simulink model "quadrotor"  (R2022b)
settings: Solver=ode4  StartTime=0.0  StopTime=120  FixedStep=0.01  RelTol=1e-3
InitFcn:
  | initial_conditions_and_parameters;
values from neighbouring files (symbols this model uses):
  ang_max = 6*pi/180    (= 0.10471975512)    [initial_conditions_and_parameters.m]
  CD = [0.018944 0.018944 0.018944]    [initial_conditions_and_parameters.m]
  data = zeros(data_len,1)    [initial_conditions_and_parameters.m]
  delay_a = 0    [initial_conditions_and_parameters.m]
  delay_sample = 0.1    [initial_conditions_and_parameters.m]
  delay_v = 0.1    [initial_conditions_and_parameters.m]
  ESC_k = 718.078    [initial_conditions_and_parameters.m]
  ESC_p = 88.448    [initial_conditions_and_parameters.m]
  f_g = [0 0 0]    [initial_conditions_and_parameters.m]
  ftau_b = [0 0 0]    [initial_conditions_and_parameters.m]
  g = 9.8    [initial_conditions_and_parameters.m]
  hM = 1.982e-7    (= 1.982e-07)    [initial_conditions_and_parameters.m]
  hT = 1.239e-5    (= 1.239e-05)    [initial_conditions_and_parameters.m]
  Ir = 3.789e-6    (= 3.789e-06)    [initial_conditions_and_parameters.m]
  Ix = 0.01    [initial_conditions_and_parameters.m]
  Iy = 0.01    [initial_conditions_and_parameters.m]
  Iz = 0.02    [initial_conditions_and_parameters.m]
  kd_phi = 70    [initial_conditions_and_parameters.m]
  kd_psi = 70    [initial_conditions_and_parameters.m]
  kd_theta = 70    [initial_conditions_and_parameters.m]
  kd_x = 1    [initial_conditions_and_parameters.m]
  kd_y = 1    [initial_conditions_and_parameters.m]
  kd_z = 1    [initial_conditions_and_parameters.m]
  Kdphi_D = 0.03    [initial_conditions_and_parameters.m]
  Kdphi_I = 0.68    [initial_conditions_and_parameters.m]
  Kdphi_P = 1    [initial_conditions_and_parameters.m]
  Kdpsi_D = 0.03    [initial_conditions_and_parameters.m]
  Kdpsi_I = 0.68    [initial_conditions_and_parameters.m]
  Kdpsi_P = 1    [initial_conditions_and_parameters.m]
  Kdtheta_D = 0.03    [initial_conditions_and_parameters.m]
  Kdtheta_I = 0.68    [initial_conditions_and_parameters.m]
  Kdtheta_P = 1    [initial_conditions_and_parameters.m]
  kp_phi = 250    [initial_conditions_and_parameters.m]
  kp_psi = 250    [initial_conditions_and_parameters.m]
  kp_theta = 250    [initial_conditions_and_parameters.m]
  kp_x = 0    [initial_conditions_and_parameters.m]
  kp_y = 0    [initial_conditions_and_parameters.m]
  kp_z = 20    [initial_conditions_and_parameters.m]
  Kvx_D = 0.15    [initial_conditions_and_parameters.m]
  Kvx_I = 0.1    [initial_conditions_and_parameters.m]
  Kvx_P = 0.3    [initial_conditions_and_parameters.m]
  Kvy_D = 0.15    [initial_conditions_and_parameters.m]
  Kvy_I = 0.1    [initial_conditions_and_parameters.m]
  Kvy_P = 0.3    [initial_conditions_and_parameters.m]
  Kvz_D = 0    [initial_conditions_and_parameters.m]
  Kvz_I = 0.1    [initial_conditions_and_parameters.m]
  Kvz_P = 1    [initial_conditions_and_parameters.m]
  LT = 0.1*sqrt(2)    [initial_conditions_and_parameters.m]
  m = 0.5    [initial_conditions_and_parameters.m]
  noise_a = 0.0005    [initial_conditions_and_parameters.m]
  noise_v = 0.0015    [initial_conditions_and_parameters.m]
  p_initial = 0    [initial_conditions_and_parameters.m]
  phi_initial = 0    [initial_conditions_and_parameters.m]
  psi_initial = 0    [initial_conditions_and_parameters.m]
  q_initial = 0    [initial_conditions_and_parameters.m]
  r_initial = 0    [initial_conditions_and_parameters.m]
  sample_a = 0.01    [initial_conditions_and_parameters.m]
  sample_v = 0.04    [initial_conditions_and_parameters.m]
  seed_delay_phi = floor(rand()*10000000)    [initial_conditions_and_parameters.m]
  seed_delay_psi = floor(rand()*10000000)    [initial_conditions_and_parameters.m]
  seed_delay_theta = floor(rand()*10000000)    [initial_conditions_and_parameters.m]
  seed_delay_vx = floor(rand()*10000000)    [initial_conditions_and_parameters.m]
  seed_delay_vy = floor(rand()*10000000)    [initial_conditions_and_parameters.m]
  seed_delay_vz = floor(rand()*10000000)    [initial_conditions_and_parameters.m]
  seed_phi = floor(rand()*10000000)    [initial_conditions_and_parameters.m]
  seed_psi = floor(rand()*10000000)    [initial_conditions_and_parameters.m]
  seed_theta = floor(rand()*10000000)    [initial_conditions_and_parameters.m]
  seed_vx = floor(rand()*10000000)    [initial_conditions_and_parameters.m]
  seed_vy = floor(rand()*10000000)    [initial_conditions_and_parameters.m]
  seed_vz = floor(rand()*10000000)    [initial_conditions_and_parameters.m]
  sweep_amp = 1    [main.m]
  T_max = 30    [initial_conditions_and_parameters.m]
  tau_x_max = 1    [initial_conditions_and_parameters.m]
  tau_y_max = 1    [initial_conditions_and_parameters.m]
  tau_z_max = 1    [initial_conditions_and_parameters.m]
  theta_initial = 0    [initial_conditions_and_parameters.m]
  u_initial = 0    [initial_conditions_and_parameters.m]
  v_initial = 0    [initial_conditions_and_parameters.m]
  w_initial = 0    [initial_conditions_and_parameters.m]
  x_g_initial = 0    [initial_conditions_and_parameters.m]
  y_g_initial = 0    [initial_conditions_and_parameters.m]
  z_g_initial = 0    [initial_conditions_and_parameters.m]
libraries: simulink x12
settings Model: Creator=Sky  LastModifiedBy=xpp
settings SolverCC: AlgebraicLoopSolver=LineSearch
settings DataIOCC: SignalLogging=off
settings DebuggingCC: InheritedTsInSrcMsg=none  TasksWithSamePriorityMsg=none  SigSpecEnsureSampleTimeMsg=none  UnconnectedInputMsg=warning  UnconnectedOutputMsg=warning  UnconnectedLineMsg=warning  UnknownTsInhSupMsg=none  SFMachineParentedDataDiag=warning  ArithmeticOperatorsInVariantConditions=warning
settings ModelReferenceCC: EnableRefExpFcnMdlSchedulingChecks=on
settings SFSimCC: SimUseLocalCustomCode=off  CustomCodeUndefinedFunction=UseInterfaceOnly
settings RTWCC: RTWUseLocalCustomCode=off  DLArmComputeVersion=19.05

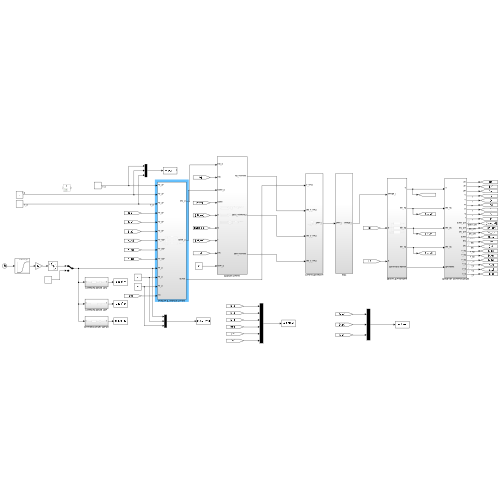
[thumbnail: Simulink's stored preview of the top-level diagram]
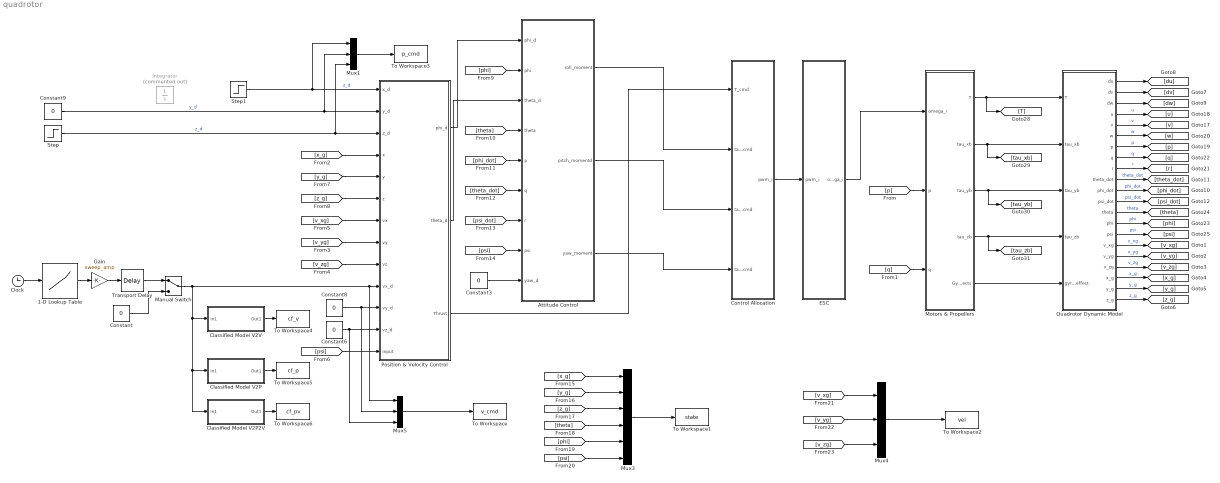
== system quadrotor ==
  1-D Lookup Table : Lookup_n-D  NumberOfTableDimensions=1  BreakpointsForDimension1=t  Table=data  InternalRulePriority=Speed  RndMeth=Simplest
  Attitude Control : Subsystem
  Classified Model V2P : Subsystem
  Classified Model V2P2V : Subsystem
  Classified Model V2V : Subsystem
  Clock : Clock
  Constant : Constant  Value=0
  Constant3 : Constant  Value=0
  Constant6 : Constant  Value=0  SampleTime=-1
  Constant8 : Constant  Value=0  SampleTime=-1
  Constant9 : Constant  Value=0  SampleTime=-1
  Control Allocation : Subsystem
  ESC : Subsystem
  Gain : Gain  Gain=sweep_amp
  Integrator : Integrator  Commented=on
  Manual Switch : ManualSwitch
  Motors & Propellers : Subsystem
  Mux1 : Mux  Inputs=3
  Mux3 : Mux  Inputs=6
  Mux4 : Mux  Inputs=3
  Mux5 : Mux  Inputs=3
  Position & Velocity Control : Subsystem
  Quadrotor Dynamic Model : Subsystem
  Step : Step  SampleTime=0
  Step1 : Step  Time=20  SampleTime=0
  To Workspace : ToWorkspace  VariableName=v_cmd  SampleTime=-1
      settings: Save2DSignal=2-D array (concatenate along first dimension)
  To Workspace1 : ToWorkspace  VariableName=state  SampleTime=-1
      settings: Save2DSignal=2-D array (concatenate along first dimension)
  To Workspace2 : ToWorkspace  VariableName=vel  SampleTime=-1
      settings: Save2DSignal=2-D array (concatenate along first dimension)
  To Workspace3 : ToWorkspace  VariableName=p_cmd  SampleTime=-1
      settings: Save2DSignal=2-D array (concatenate along first dimension)
  To Workspace4 : ToWorkspace  VariableName=cf_v  SampleTime=-1
      settings: Save2DSignal=2-D array (concatenate along first dimension)
  To Workspace5 : ToWorkspace  VariableName=cf_p  SampleTime=-1
      settings: Save2DSignal=2-D array (concatenate along first dimension)
  To Workspace6 : ToWorkspace  VariableName=cf_pv  SampleTime=-1
      settings: Save2DSignal=2-D array (concatenate along first dimension)
  Transport Delay : TransportDelay  DelayTime=20  BufferSize=4096
  wires:
  [q] -> Motors & Propellers/3(q)
  [p] -> Motors & Propellers/2(p)
  Motors & Propellers/1(T) -> Quadrotor Dynamic Model/1(T), [T]
  Motors & Propellers/2(tau_xb) -> Quadrotor Dynamic Model/2(tau_xb), [tau_xb]
  Motors & Propellers/3(tau_yb) -> Quadrotor Dynamic Model/3(tau_yb), [tau_yb]
  Motors & Propellers/4(tau_zb) -> Quadrotor Dynamic Model/4(tau_zb), [tau_zb]
  Quadrotor Dynamic Model/3(dw) -> [dw]
  Quadrotor Dynamic Model/8(q) -> [q]  "q"
  Quadrotor Dynamic Model/12(psi_dot) -> [psi_dot]  "psi_dot"
  Quadrotor Dynamic Model/18(v_zg) -> [v_zg]  "v_zg"
  Quadrotor Dynamic Model/5(v) -> [v]  "v"
  Quadrotor Dynamic Model/9(r) -> [r]  "r"
  Quadrotor Dynamic Model/11(phi_dot) -> [phi_dot]  "phi_dot"
  Quadrotor Dynamic Model/1(du) -> [du]
  Quadrotor Dynamic Model/19(x_g) -> [x_g]  "x_g"
  Quadrotor Dynamic Model/20(y_g) -> [y_g]  "y_g"
  Quadrotor Dynamic Model/16(v_xg) -> [v_xg]  "v_xg"
  Quadrotor Dynamic Model/15(psi) -> [psi]  "psi"
  Quadrotor Dynamic Model/4(u) -> [u]  "u"
  Quadrotor Dynamic Model/13(theta) -> [theta]  "theta"
  Quadrotor Dynamic Model/17(v_yg) -> [v_yg]  "v_yg"
  Quadrotor Dynamic Model/14(phi) -> [phi]  "phi"
  Quadrotor Dynamic Model/21(z_g) -> [z_g]  "z_g"
  Quadrotor Dynamic Model/6(w) -> [w]  "w"
  Quadrotor Dynamic Model/7(p) -> [p]  "p"
  Quadrotor Dynamic Model/2(dv) -> [dv]
  Quadrotor Dynamic Model/10(theta_dot) -> [theta_dot]  "theta_dot"
  [x_g] -> Position & Velocity Control/4(x)
  [v_yg] -> Position & Velocity Control/8(vy)
  [v_zg] -> Position & Velocity Control/9(vz)
  [v_xg] -> Position & Velocity Control/7(vx)
  [y_g] -> Position & Velocity Control/5(y)
  [z_g] -> Position & Velocity Control/6(z)
  Position & Velocity Control/1(phi_d) -> Attitude Control/1(phi_d)
  Position & Velocity Control/2(theta_d) -> Attitude Control/3(theta_d)
  [phi] -> Attitude Control/2(phi)
  [theta] -> Attitude Control/4(theta)
  [phi_dot] -> Attitude Control/5(p)
  [theta_dot] -> Attitude Control/6(q)
  [psi_dot] -> Attitude Control/7(r)
  [psi] -> Attitude Control/8(psi)
  Constant9/1 -> Mux1/2, Position & Velocity Control/2(y_d)  "y_d"
  Step/1 -> Mux1/3, Position & Velocity Control/3(z_d)  "z_d"
  Constant3/1 -> Attitude Control/9(yaw_d)
  Control Allocation/1(pwm_i) -> ESC/1(pwm_i)
  ESC/1(omega_i) -> Motors & Propellers/1(omega_i)
  Attitude Control/3(yaw_moment) -> Control Allocation/4(tau_z_cmd)
  Attitude Control/1(roll_moment) -> Control Allocation/2(tau_x_cmd)
  Attitude Control/2(pitch_momentd) -> Control Allocation/3(tau_y_cmd)
  Position & Velocity Control/3(Thrust) -> Control Allocation/1(T_cmd)
  Motors & Propellers/5(Gyroscopic effects) -> Quadrotor Dynamic Model/5(gyroeffect)
  Mux3/1 -> To Workspace1/1
  [x_g] -> Mux3/1
  [y_g] -> Mux3/2
  [z_g] -> Mux3/3
  [theta] -> Mux3/4
  [phi] -> Mux3/5
  [psi] -> Mux3/6
  Mux5/1 -> To Workspace/1
  Constant6/1 -> Mux5/3, Position & Velocity Control/12(vz_d)
  Constant8/1 -> Mux5/2, Position & Velocity Control/11(vy_d)
  Clock/1 -> 1-D Lookup Table/1
  Mux4/1 -> To Workspace2/1
  [v_zg] -> Mux4/3
  [v_yg] -> Mux4/2
  [v_xg] -> Mux4/1
  Step1/1 -> Mux1/1, Position & Velocity Control/1(x_d)  "z_d"
  Mux1/1 -> To Workspace3/1
  [psi] -> Position & Velocity Control/13(Input)
  Manual Switch/1 -> Classified Model V2P2V/1(In1), Classified Model V2P/1(In1), Classified Model V2V/1(In1), Mux5/1, Position & Velocity Control/10(vx_d)
  Transport Delay/1 -> Manual Switch/1
  Constant/1 -> Manual Switch/2
  Classified Model V2V/1(Out1) -> To Workspace4/1
  Classified Model V2P/1(Out1) -> To Workspace5/1
  Classified Model V2P2V/1(Out1) -> To Workspace6/1
  Gain/1 -> Transport Delay/1
  1-D Lookup Table/1 -> Gain/1

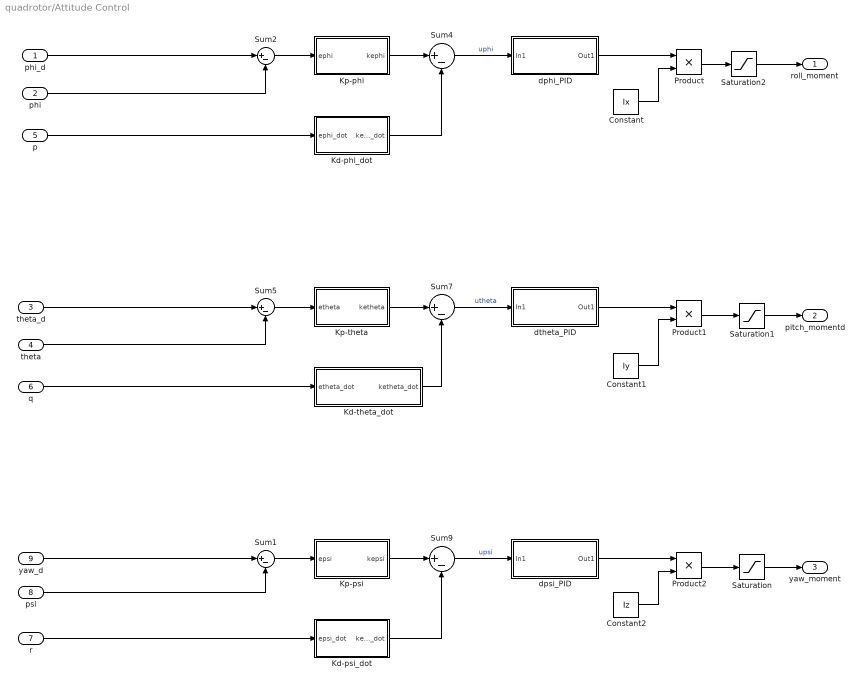
== system quadrotor/Attitude Control ==
  phi_d : Inport
  phi : Inport  Port=2
  theta_d : Inport  Port=3
  theta : Inport  Port=4
  p : Inport  Port=5
  q : Inport  Port=6
  r : Inport  Port=7
  psi : Inport  Port=8
  yaw_d : Inport  Port=9
  Constant : Constant  Value=Ix
  Constant1 : Constant  Value=Iy
  Constant2 : Constant  Value=Iz
  Kd-phi_dot : Subsystem
  Kd-psi_dot : Subsystem
  Kd-theta_dot : Subsystem
  Kp-phi : Subsystem
  Kp-psi : Subsystem
  Kp-theta : Subsystem
  Product : Product  OutMin=[-1]  OutMax=[1]
  Product1 : Product  OutMin=[-1]  OutMax=[1]
  Product2 : Product  OutMin=[-1]  OutMax=[1]
  Saturation : Saturate  UpperLimit=tau_z_max  LowerLimit=-tau_z_max
  Saturation1 : Saturate  UpperLimit=tau_y_max  LowerLimit=-tau_y_max
  Saturation2 : Saturate  UpperLimit=tau_x_max  LowerLimit=-tau_x_max
  Sum{1..2,4..5,7,9} (6 alike) : Sum  Inputs=|+-
  dphi_PID : Subsystem
  dpsi_PID : Subsystem
  dtheta_PID : Subsystem
  roll_moment : Outport
  pitch_momentd : Outport  Port=2
  yaw_moment : Outport  Port=3
  wires:
  r/1 -> Kd-psi_dot/1(epsi_dot)
  Sum1/1 -> Kp-psi/1(epsi)
  p/1 -> Kd-phi_dot/1(ephi_dot)
  Sum2/1 -> Kp-phi/1(ephi)
  phi_d/1 -> Sum2/1
  Kd-phi_dot/1(kephi_dot) -> Sum4/2
  q/1 -> Kd-theta_dot/1(etheta_dot)
  Sum5/1 -> Kp-theta/1(etheta)
  theta_d/1 -> Sum5/1
  Kd-theta_dot/1(ketheta_dot) -> Sum7/2
  yaw_d/1 -> Sum1/1
  Constant/1 -> Product/2
  Product/1 -> Saturation2/1
  Product1/1 -> Saturation1/1
  Constant1/1 -> Product1/2
  Product2/1 -> Saturation/1
  Constant2/1 -> Product2/2
  Saturation/1 -> yaw_moment/1
  Saturation1/1 -> pitch_momentd/1
  Saturation2/1 -> roll_moment/1
  Kp-phi/1(kephi) -> Sum4/1
  Kp-theta/1(ketheta) -> Sum7/1
  Kp-psi/1(kepsi) -> Sum9/1
  Kd-psi_dot/1(kepsi_dot) -> Sum9/2
  dphi_PID/1(Out1) -> Product/1
  Sum4/1 -> dphi_PID/1(In1)  "uphi"
  Sum7/1 -> dtheta_PID/1(In1)  "utheta"
  dtheta_PID/1(Out1) -> Product1/1
  Sum9/1 -> dpsi_PID/1(In1)  "upsi"
  dpsi_PID/1(Out1) -> Product2/1
  phi/1 -> Sum2/2
  theta/1 -> Sum5/2
  psi/1 -> Sum1/2

== system quadrotor/Classified Model V2P ==
  In1 : Inport
  Transfer Fcn : TransferFcn  Numerator=[2.218]  Denominator=[1 2.1565 0.0006694]
  Transport Delay : TransportDelay  DelayTime=0.06
  Out1 : Outport
  wires:
  Transfer Fcn/1 -> Transport Delay/1
  In1/1 -> Transfer Fcn/1
  Transport Delay/1 -> Out1/1

== system quadrotor/Classified Model V2P2V ==
  In1 : Inport
  Transfer Fcn : TransferFcn  Numerator=[2.218]  Denominator=[1 2.16]
  Transport Delay : TransportDelay  DelayTime=0.06
  Out1 : Outport
  wires:
  Transfer Fcn/1 -> Transport Delay/1
  In1/1 -> Transfer Fcn/1
  Transport Delay/1 -> Out1/1

== system quadrotor/Classified Model V2V ==
  In1 : Inport
  Transfer Fcn : TransferFcn  Numerator=[2.135]  Denominator=[1 2.016]
  Transport Delay : TransportDelay  DelayTime=0.06
  Out1 : Outport
  wires:
  In1/1 -> Transfer Fcn/1
  Transfer Fcn/1 -> Transport Delay/1
  Transport Delay/1 -> Out1/1

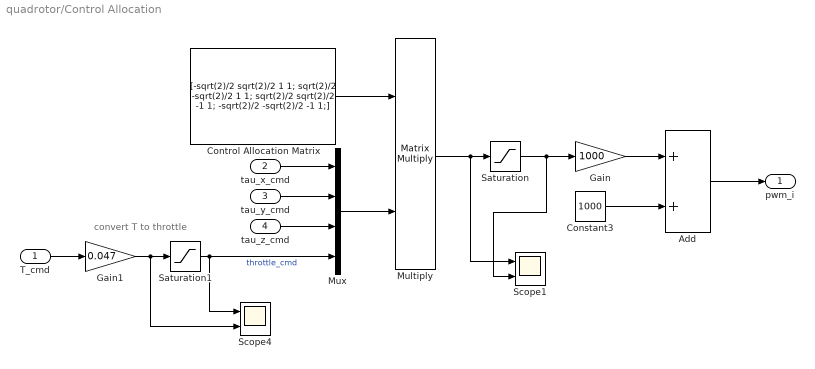
== system quadrotor/Control Allocation ==
  note: convert T to throttle
  T_cmd : Inport
  tau_x_cmd : Inport  Port=2
  tau_y_cmd : Inport  Port=3
  tau_z_cmd : Inport  Port=4
  Add : Sum
  Constant3 : Constant  Value=1000
  Control Allocation Matrix : Constant  Value="[-sqrt(2)/2  sqrt(2)/2  1 1; sqrt(2)/2 -sqrt(2)/2  1 1; sqrt(2)/2  sqrt(2)/2 -1 1; -sqrt(2)/2 -sqrt(2)/2 -1 1;]"
  Gain : Gain  Gain=1000  OutDataTypeStr=Inherit: Same as input
  Gain1 : Gain  Gain=0.047
  Multiply : Product  Multiplication=Matrix(*)  OutDataTypeStr=Inherit: Same as first input
  Mux : Mux
  Saturation : Saturate  UpperLimit=1  LowerLimit=0
  Saturation1 : Saturate  UpperLimit=1  LowerLimit=0
  Scope1 : Scope  NumInputPorts=2
  Scope4 : Scope  NumInputPorts=2
  pwm_i : Outport  VectorParamsAs1DForOutWhenUnconnected=off
  wires:
  Constant3/1 -> Add/2
  Saturation/1 -> Scope1/2, Gain/1
  Saturation1/1 -> Scope4/1, Mux/4  "throttle_cmd"
  tau_y_cmd/1 -> Mux/2
  Add/1 -> pwm_i/1
  Multiply/1 -> Scope1/1, Saturation/1
  Gain/1 -> Add/1
  tau_x_cmd/1 -> Mux/1
  tau_z_cmd/1 -> Mux/3
  Mux/1 -> Multiply/2
  Control Allocation Matrix/1 -> Multiply/1
  Gain1/1 -> Scope4/2, Saturation1/1
  T_cmd/1 -> Gain1/1

== system quadrotor/ESC ==
  pwm_i : Inport
  Add : Sum  AccumDataTypeStr=double
  Constant : Constant  Value=ESC_p
  Constant3 : Constant  Value=1000  OutDataTypeStr=double
  Gain : Gain  Gain=0.001  OutDataTypeStr=Inherit: Same as input
  Gain1 : Gain  Gain=ESC_k  OutDataTypeStr=Inherit: Same as input
  Saturation : Saturate  UpperLimit=2000  LowerLimit=1000
  Sum : Sum  Inputs=|+-
  omega_i : Outport  VectorParamsAs1DForOutWhenUnconnected=off
  wires:
  Constant3/1 -> Sum/2
  pwm_i/1 -> Saturation/1
  Saturation/1 -> Sum/1
  Sum/1 -> Gain/1
  Constant/1 -> Add/2
  Gain/1 -> Gain1/1
  Gain1/1 -> Add/1
  Add/1 -> omega_i/1

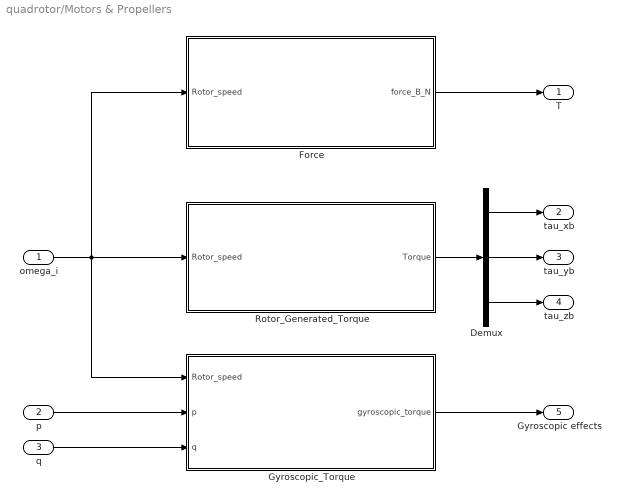
== system quadrotor/Motors & Propellers ==
  omega_i : Inport
  p : Inport  Port=2
  q : Inport  Port=3
  Demux : Demux  Outputs=3
  Force : Subsystem
  Gyroscopic_Torque : Subsystem
  Rotor_Generated_Torque : Subsystem
  T : Outport  VectorParamsAs1DForOutWhenUnconnected=off
  tau_xb : Outport  Port=2  VectorParamsAs1DForOutWhenUnconnected=off
  tau_yb : Outport  Port=3  VectorParamsAs1DForOutWhenUnconnected=off
  tau_zb : Outport  Port=4  VectorParamsAs1DForOutWhenUnconnected=off
  Gyroscopic effects : Outport  Port=5  VectorParamsAs1DForOutWhenUnconnected=off
  wires:
  Rotor_Generated_Torque/1(Torque) -> Demux/1
  p/1 -> Gyroscopic_Torque/2(p)
  omega_i/1 -> Force/1(Rotor_speed), Gyroscopic_Torque/1(Rotor_speed), Rotor_Generated_Torque/1(Rotor_speed)
  Force/1(force_B_N) -> T/1
  Gyroscopic_Torque/1(gyroscopic_torque) -> Gyroscopic effects/1
  Demux/1 -> tau_xb/1
  Demux/2 -> tau_yb/1
  Demux/3 -> tau_zb/1
  q/1 -> Gyroscopic_Torque/3(q)

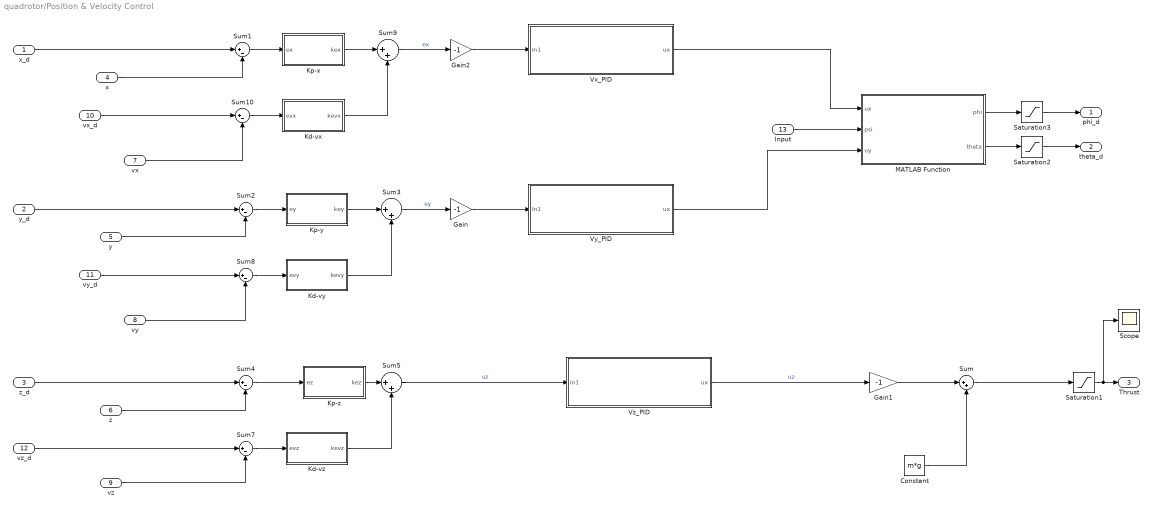
== system quadrotor/Position & Velocity Control ==
  x_d : Inport
  y_d : Inport  Port=2
  z_d : Inport  Port=3
  x : Inport  Port=4
  y : Inport  Port=5
  z : Inport  Port=6
  vx : Inport  Port=7
  vy : Inport  Port=8
  vz : Inport  Port=9
  vx_d : Inport  Port=10
  vy_d : Inport  Port=11
  vz_d : Inport  Port=12
  Input : Inport  Port=13
  Constant : Constant  Value=m*g
  Gain : Gain  Gain=-1
  Gain1 : Gain  Gain=-1
  Gain2 : Gain  Gain=-1
  Kd-vx : Subsystem
  Kd-vy : Subsystem
  Kd-vz : Subsystem
  Kp-x : Subsystem
  Kp-y : Subsystem
  Kp-z : Subsystem
  MATLAB Function : MATLAB Function  TreatAsAtomicUnit=on
  Saturation1 : Saturate  UpperLimit=15  LowerLimit=-T_max
  Saturation2 : Saturate  UpperLimit=ang_max  LowerLimit=-ang_max
  Saturation3 : Saturate  UpperLimit=ang_max  LowerLimit=-ang_max  LinearizeAsGain=off
  Scope : Scope
  Sum{,3,5,9} (4 alike) : Sum  Inputs=|++
  Sum{1..2,4,7..8,10} (6 alike) : Sum  Inputs=|+-
  Vx_PID : Subsystem
  Vy_PID : Subsystem
  Vz_PID : Subsystem
  phi_d : Outport
  theta_d : Outport  Port=2
  Thrust : Outport  Port=3  OutMin=[-30]  OutMax=[0]
  wires:
  Sum4/1 -> Kp-z/1(ez)
  z/1 -> Sum4/2
  z_d/1 -> Sum4/1
  Sum7/1 -> Kd-vz/1(evz)
  Kp-z/1(kez) -> Sum5/1
  Kd-vz/1(kevz) -> Sum5/2
  Sum8/1 -> Kd-vy/1(evy)
  Kp-y/1(key) -> Sum3/1
  y/1 -> Sum2/2
  Kd-vy/1(kevy) -> Sum3/2
  Sum2/1 -> Kp-y/1(ey)
  y_d/1 -> Sum2/1
  Kd-vx/1(kevx) -> Sum9/2
  Sum1/1 -> Kp-x/1(ex)
  Sum10/1 -> Kd-vx/1(evx)
  x/1 -> Sum1/2
  x_d/1 -> Sum1/1
  Sum5/1 -> Vz_PID/1(In1)  "uz"
  Vz_PID/1(ux) -> Gain1/1  "uz"
  Saturation1/1 -> Scope/1, Thrust/1
  vz_d/1 -> Sum7/1
  Kp-x/1(kex) -> Sum9/1
  vy_d/1 -> Sum8/1
  MATLAB Function/2(theta) -> Saturation2/1
  MATLAB Function/1(phi) -> Saturation3/1
  Vx_PID/1(ux) -> MATLAB Function/1(ux)
  Input/1 -> MATLAB Function/2(psi)
  Sum3/1 -> Gain/1  "ey"
  Saturation3/1 -> phi_d/1
  Saturation2/1 -> theta_d/1
  Sum9/1 -> Gain2/1  "ex"
  Vy_PID/1(ux) -> MATLAB Function/3(uy)
  Gain/1 -> Vy_PID/1(In1)
  Gain2/1 -> Vx_PID/1(In1)
  vx_d/1 -> Sum10/1
  vx/1 -> Sum10/2
  vy/1 -> Sum8/2
  vz/1 -> Sum7/2
  Gain1/1 -> Sum/1
  Sum/1 -> Saturation1/1
  Constant/1 -> Sum/2

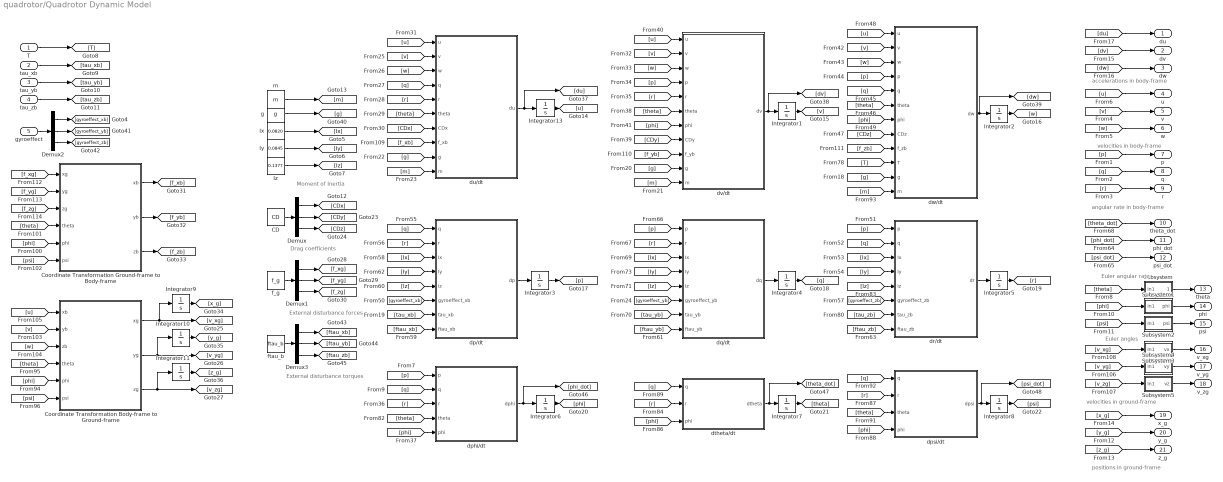
== system quadrotor/Quadrotor Dynamic Model ==
  note: velocities in body-frame
  note: accelerations in body-frame
  note: Moment of Inertia
  note: Drag coefficients
  note: External disturbance forces
  note: External disturbance torques
  note: angular rate in body-frame
  note: Euler angular rate
  note: Euler angles
  note: velocities in ground-frame
  note: positions in ground-frame
  T : Inport
  tau_xb : Inport  Port=2
  tau_yb : Inport  Port=3
  tau_zb : Inport  Port=4
  gyroeffect : Inport  Port=5
  CD : Constant  Value=CD
  Coordinate Transformation Body-frame to Ground-frame : MATLAB Function  TreatAsAtomicUnit=on
  Coordinate Transformation Ground-frame to Body-frame : MATLAB Function  TreatAsAtomicUnit=on
  Demux{,1..3} (4 alike) : Demux  Outputs=3
  Integrator1 : Integrator  InitialCondition=v_initial
  Integrator10 : Integrator  InitialCondition=y_g_initial
  Integrator11 : Integrator  InitialCondition=z_g_initial
  Integrator13 : Integrator  InitialCondition=u_initial
  Integrator2 : Integrator  InitialCondition=w_initial
  Integrator3 : Integrator  InitialCondition=p_initial
  Integrator4 : Integrator  InitialCondition=q_initial
  Integrator5 : Integrator  InitialCondition=r_initial
  Integrator6 : Integrator  InitialCondition=phi_initial
  Integrator7 : Integrator  InitialCondition=theta_initial
  Integrator8 : Integrator  InitialCondition=psi_initial
  Integrator9 : Integrator  InitialCondition=x_g_initial
  Ix : Constant  Value=0.0820
  Iy : Constant  Value=0.0845
  Iz : Constant  Value=0.1377
  Subsystem : Subsystem
  Subsystem1 : Subsystem
  Subsystem2 : Subsystem
  Subsystem3 : Subsystem
  Subsystem4 : Subsystem
  Subsystem5 : Subsystem
  dp/dt : MATLAB Function  TreatAsAtomicUnit=on
  dphi/dt : MATLAB Function  TreatAsAtomicUnit=on
  dpsi/dt : MATLAB Function  TreatAsAtomicUnit=on
  dq/dt : MATLAB Function  TreatAsAtomicUnit=on
  dr/dt : MATLAB Function  TreatAsAtomicUnit=on
  dtheta/dt : MATLAB Function  TreatAsAtomicUnit=on
  du/dt : MATLAB Function  TreatAsAtomicUnit=on
  dv/dt : MATLAB Function  TreatAsAtomicUnit=on
  dw/dt : MATLAB Function  TreatAsAtomicUnit=on
  f_g : Constant  Value=f_g
  ftau_b : Constant  Value=ftau_b
  g : Constant  Value=g
  m : Constant  Value=m
  du : Outport  VectorParamsAs1DForOutWhenUnconnected=off
  dv : Outport  Port=2  VectorParamsAs1DForOutWhenUnconnected=off
  dw : Outport  Port=3  VectorParamsAs1DForOutWhenUnconnected=off
  u : Outport  Port=4  VectorParamsAs1DForOutWhenUnconnected=off
  v : Outport  Port=5  VectorParamsAs1DForOutWhenUnconnected=off
  w : Outport  Port=6  VectorParamsAs1DForOutWhenUnconnected=off
  p : Outport  Port=7  VectorParamsAs1DForOutWhenUnconnected=off
  q : Outport  Port=8  VectorParamsAs1DForOutWhenUnconnected=off
  r : Outport  Port=9  VectorParamsAs1DForOutWhenUnconnected=off
  theta_dot : Outport  Port=10  VectorParamsAs1DForOutWhenUnconnected=off
  phi_dot : Outport  Port=11  VectorParamsAs1DForOutWhenUnconnected=off
  psi_dot : Outport  Port=12  VectorParamsAs1DForOutWhenUnconnected=off
  theta : Outport  Port=13  VectorParamsAs1DForOutWhenUnconnected=off
  phi : Outport  Port=14  VectorParamsAs1DForOutWhenUnconnected=off
  psi : Outport  Port=15  VectorParamsAs1DForOutWhenUnconnected=off
  v_xg : Outport  Port=16  VectorParamsAs1DForOutWhenUnconnected=off
  v_yg : Outport  Port=17  VectorParamsAs1DForOutWhenUnconnected=off
  v_zg : Outport  Port=18  VectorParamsAs1DForOutWhenUnconnected=off
  x_g : Outport  Port=19  VectorParamsAs1DForOutWhenUnconnected=off
  y_g : Outport  Port=20  VectorParamsAs1DForOutWhenUnconnected=off
  z_g : Outport  Port=21  VectorParamsAs1DForOutWhenUnconnected=off
  wires:
  Ix/1 -> [Ix]
  Iy/1 -> [Iy]
  Iz/1 -> [Iz]
  T/1 -> [T]
  tau_xb/1 -> [tau_xb]
  tau_yb/1 -> [tau_yb]
  tau_zb/1 -> [tau_zb]
  CD/1 -> Demux/1
  m/1 -> [m]
  [v] -> du/dt/2(v)
  [w] -> du/dt/3(w)
  [q] -> du/dt/4(q)
  [r] -> du/dt/5(r)
  [theta] -> du/dt/6(theta)
  [CDx] -> du/dt/7(CDx)
  [u] -> du/dt/1(u)
  du/dt/1(du) -> [du], Integrator13/1
  Integrator13/1 -> [u]
  [v] -> dv/dt/2(v)
  [w] -> dv/dt/3(w)
  [p] -> dv/dt/4(p)
  [r] -> dv/dt/5(r)
  [theta] -> dv/dt/6(theta)
  [CDy] -> dv/dt/8(CDy)
  [u] -> dv/dt/1(u)
  dv/dt/1(dv) -> [dv], Integrator1/1
  Integrator1/1 -> [v]
  [phi] -> dv/dt/7(phi)
  [v] -> dw/dt/2(v)
  [w] -> dw/dt/3(w)
  [p] -> dw/dt/4(p)
  [q] -> dw/dt/5(q)
  [theta] -> dw/dt/6(theta)
  [CDz] -> dw/dt/8(CDz)
  [u] -> dw/dt/1(u)
  dw/dt/1(dw) -> [dw], Integrator2/1
  Integrator2/1 -> [w]
  [phi] -> dw/dt/7(phi)
  dp/dt/1(dp) -> Integrator3/1
  Integrator3/1 -> [p]
  [gyroeffect_xb] -> dp/dt/6(gyroeffect_xb)
  [q] -> dp/dt/1(q)
  [r] -> dp/dt/2(r)
  [Iz] -> dp/dt/5(Iz)
  [Ix] -> dp/dt/3(Ix)
  [Iy] -> dp/dt/4(Iy)
  dq/dt/1(dq) -> Integrator4/1
  Integrator4/1 -> [q]
  [p] -> dq/dt/1(p)
  [r] -> dq/dt/2(r)
  [Iz] -> dq/dt/5(Iz)
  [Ix] -> dq/dt/3(Ix)
  [tau_yb] -> dq/dt/7(tau_yb)
  [Iy] -> dq/dt/4(Iy)
  dr/dt/1(dr) -> Integrator5/1
  Integrator5/1 -> [r]
  [tau_zb] -> dr/dt/7(tau_zb)
  [Iz] -> dr/dt/5(Iz)
  dphi/dt/1(dphi) -> [phi_dot], Integrator6/1
  Integrator6/1 -> [phi]
  [p] -> dphi/dt/1(p)
  [q] -> dphi/dt/2(q)
  [r] -> dphi/dt/3(r)
  [theta] -> dphi/dt/4(theta)
  [phi] -> dphi/dt/5(phi)
  dtheta/dt/1(dtheta) -> [theta_dot], Integrator7/1
  Integrator7/1 -> [theta]
  [q] -> dtheta/dt/1(q)
  [r] -> dtheta/dt/2(r)
  [phi] -> dtheta/dt/3(phi)
  dpsi/dt/1(dpsi) -> [psi_dot], Integrator8/1
  Integrator8/1 -> [psi]
  [q] -> dpsi/dt/1(q)
  [r] -> dpsi/dt/2(r)
  [theta] -> dpsi/dt/3(theta)
  [phi] -> dpsi/dt/4(phi)
  Demux/1 -> [CDx]
  Demux/2 -> [CDy]
  Demux/3 -> [CDz]
  [u] -> u/1
  [v] -> v/1
  [w] -> w/1
  [p] -> p/1
  [q] -> q/1
  [r] -> r/1
  [T] -> dw/dt/10(T)
  [m] -> dw/dt/12(m)
  [theta] -> Coordinate Transformation Body-frame to Ground-frame/4(theta)
  [phi] -> Coordinate Transformation Body-frame to Ground-frame/5(phi)
  [psi] -> Coordinate Transformation Body-frame to Ground-frame/6(psi)
  [theta] -> Coordinate Transformation Ground-frame to Body-frame/4(theta)
  [phi] -> Coordinate Transformation Ground-frame to Body-frame/5(phi)
  [psi] -> Coordinate Transformation Ground-frame to Body-frame/6(psi)
  [u] -> Coordinate Transformation Body-frame to Ground-frame/1(xb)
  [v] -> Coordinate Transformation Body-frame to Ground-frame/2(yb)
  [w] -> Coordinate Transformation Body-frame to Ground-frame/3(zb)
  Coordinate Transformation Body-frame to Ground-frame/1(xg) -> Integrator9/1, [v_xg]
  Coordinate Transformation Body-frame to Ground-frame/2(yg) -> Integrator10/1, [v_yg]
  Coordinate Transformation Body-frame to Ground-frame/3(zg) -> Integrator11/1, [v_zg]
  f_g/1 -> Demux1/1
  Demux1/1 -> [f_xg]
  Demux1/2 -> [f_yg]
  Demux1/3 -> [f_zg]
  Coordinate Transformation Ground-frame to Body-frame/1(xb) -> [f_xb]
  Coordinate Transformation Ground-frame to Body-frame/2(yb) -> [f_yb]
  Coordinate Transformation Ground-frame to Body-frame/3(zb) -> [f_zb]
  [f_xb] -> du/dt/8(f_xb)
  [f_yb] -> dv/dt/9(f_yb)
  [f_zb] -> dw/dt/9(f_zb)
  [f_xg] -> Coordinate Transformation Ground-frame to Body-frame/1(xg)
  [f_yg] -> Coordinate Transformation Ground-frame to Body-frame/2(yg)
  [f_zg] -> Coordinate Transformation Ground-frame to Body-frame/3(zg)
  Integrator9/1 -> [x_g]
  Integrator10/1 -> [y_g]
  Integrator11/1 -> [z_g]
  [du] -> du/1
  [dv] -> dv/1
  [dw] -> dw/1
  g/1 -> [g]
  [g] -> dw/dt/11(g)
  [g] -> dv/dt/10(g)
  [m] -> dv/dt/11(m)
  [m] -> du/dt/10(m)
  [g] -> du/dt/9(g)
  Demux2/3 -> [gyroeffect_zb]
  Demux2/2 -> [gyroeffect_yb]
  Demux2/1 -> [gyroeffect_xb]
  gyroeffect/1 -> Demux2/1
  [tau_xb] -> dp/dt/7(tau_xb)
  [gyroeffect_yb] -> dq/dt/6(gyroeffect_yb)
  [Iy] -> dr/dt/4(Iy)
  [p] -> dr/dt/1(p)
  [q] -> dr/dt/2(q)
  [Ix] -> dr/dt/3(Ix)
  [gyroeffect_zb] -> dr/dt/6(gyroeffect_zb)
  Demux3/3 -> [ftau_zb]
  Demux3/1 -> [ftau_xb]
  Demux3/2 -> [ftau_yb]
  ftau_b/1 -> Demux3/1
  [ftau_xb] -> dp/dt/8(ftau_xb)
  [ftau_yb] -> dq/dt/8(ftau_yb)
  [ftau_zb] -> dr/dt/8(ftau_zb)
  [theta_dot] -> theta_dot/1
  [phi_dot] -> phi_dot/1
  [psi_dot] -> psi_dot/1
  [v_xg] -> Subsystem3/1(In1)
  [v_yg] -> Subsystem4/1(In1)
  [v_zg] -> Subsystem5/1(In1)
  [theta] -> Subsystem/1(In1)
  [phi] -> Subsystem1/1(In1)
  [psi] -> Subsystem2/1(In1)
  Subsystem/1(theta) -> theta/1
  Subsystem1/1(phi) -> phi/1
  Subsystem2/1(psi) -> psi/1
  Subsystem3/1(vx) -> v_xg/1
  Subsystem4/1(vy) -> v_yg/1
  [x_g] -> x_g/1
  [y_g] -> y_g/1
  Subsystem5/1(vz) -> v_zg/1
  [z_g] -> z_g/1

== system quadrotor/Attitude Control/Kd-phi_dot ==
  ephi_dot : Inport
  Gain : Gain  Gain=kd_phi
  kephi_dot : Outport
  wires:
  ephi_dot/1 -> Gain/1
  Gain/1 -> kephi_dot/1

== system quadrotor/Attitude Control/Kd-psi_dot ==
  epsi_dot : Inport
  Gain : Gain  Gain=kd_psi
  kepsi_dot : Outport
  wires:
  epsi_dot/1 -> Gain/1
  Gain/1 -> kepsi_dot/1

== system quadrotor/Attitude Control/Kd-theta_dot ==
  etheta_dot : Inport
  Gain : Gain  Gain=kd_theta
  ketheta_dot : Outport
  wires:
  etheta_dot/1 -> Gain/1
  Gain/1 -> ketheta_dot/1

== system quadrotor/Attitude Control/Kp-phi ==
  ephi : Inport
  Gain : Gain  Gain=kp_phi
  kephi : Outport
  wires:
  ephi/1 -> Gain/1
  Gain/1 -> kephi/1

== system quadrotor/Attitude Control/Kp-psi ==
  epsi : Inport
  Gain : Gain  Gain=kp_psi
  kepsi : Outport
  wires:
  epsi/1 -> Gain/1
  Gain/1 -> kepsi/1

== system quadrotor/Attitude Control/Kp-theta ==
  etheta : Inport
  Gain : Gain  Gain=kp_theta
  ketheta : Outport
  wires:
  etheta/1 -> Gain/1
  Gain/1 -> ketheta/1

== system quadrotor/Attitude Control/dphi_PID ==
  In1 : Inport
  Derivative1 : Derivative  CoefficientInTFapproximation=T_d_angle_rate
  Gain6 : Gain  Gain=Kdphi_P
  Gain7 : Gain  Gain=Kdphi_I
  Gain8 : Gain  Gain=Kdphi_D
  Integrator1 : Integrator  LimitOutput=on  UpperSaturationLimit=0.4  LowerSaturationLimit=-0.4
  Sum11 : Sum  Inputs=+++
  Out1 : Outport
  wires:
  In1/1 -> Gain6/1  "ex"
  Gain6/1 -> Sum11/2, Gain8/1, Gain7/1
  Integrator1/1 -> Sum11/1
  Gain8/1 -> Derivative1/1
  Derivative1/1 -> Sum11/3
  Gain7/1 -> Integrator1/1
  Sum11/1 -> Out1/1

== system quadrotor/Attitude Control/dpsi_PID ==
  In1 : Inport
  Derivative1 : Derivative  CoefficientInTFapproximation=T_d_angle_rate
  Gain6 : Gain  Gain=Kdpsi_P
  Gain7 : Gain  Gain=Kdpsi_I
  Gain8 : Gain  Gain=Kdpsi_D
  Integrator1 : Integrator  LimitOutput=on  UpperSaturationLimit=0.4  LowerSaturationLimit=-0.4
  Sum11 : Sum  Inputs=+++
  Out1 : Outport
  wires:
  In1/1 -> Gain6/1  "ex"
  Gain6/1 -> Sum11/2, Gain8/1, Gain7/1
  Integrator1/1 -> Sum11/1
  Gain8/1 -> Derivative1/1
  Derivative1/1 -> Sum11/3
  Gain7/1 -> Integrator1/1
  Sum11/1 -> Out1/1

== system quadrotor/Attitude Control/dtheta_PID ==
  In1 : Inport
  Derivative1 : Derivative  CoefficientInTFapproximation=T_d_angle_rate
  Gain6 : Gain  Gain=Kdtheta_P
  Gain7 : Gain  Gain=Kdtheta_I
  Gain8 : Gain  Gain=Kdtheta_D
  Integrator1 : Integrator  LimitOutput=on  UpperSaturationLimit=0.4  LowerSaturationLimit=-0.4
  Sum11 : Sum  Inputs=+++
  Out1 : Outport
  wires:
  In1/1 -> Gain6/1  "ex"
  Gain6/1 -> Sum11/2, Gain8/1, Gain7/1
  Integrator1/1 -> Sum11/1
  Gain8/1 -> Derivative1/1
  Derivative1/1 -> Sum11/3
  Gain7/1 -> Integrator1/1
  Sum11/1 -> Out1/1

== system quadrotor/Motors & Propellers/Force ==
  Rotor_speed : Inport
  Gain : Gain  OutDataTypeStr=Inherit: Same as input
  Multiply : Product  OutDataTypeStr=Inherit: Same as first input
  Square : Math  Operator=square  SignedPower=on  OutDataTypeStr=double
  Sum of Elements : Sum  Inputs=+  OutDataTypeStr=Inherit: Same as first input
  cT : Constant  Value=hT
  force_B_N : Outport  VectorParamsAs1DForOutWhenUnconnected=off
  wires:
  Multiply/1 -> Sum of Elements/1
  Square/1 -> Multiply/1
  cT/1 -> Multiply/2
  Rotor_speed/1 -> Square/1
  Gain/1 -> force_B_N/1
  Sum of Elements/1 -> Gain/1

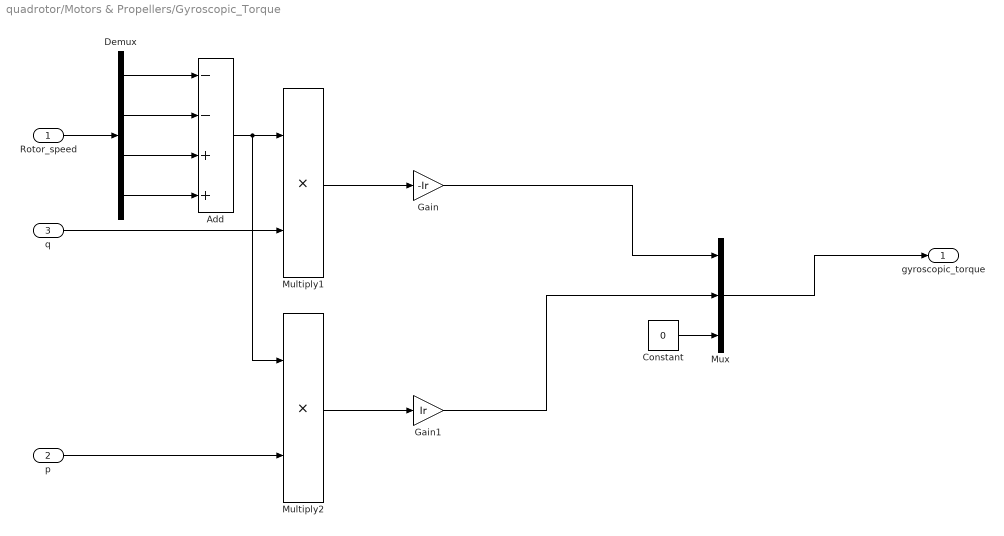
== system quadrotor/Motors & Propellers/Gyroscopic_Torque ==
  Rotor_speed : Inport
  p : Inport  Port=2
  q : Inport  Port=3
  Add : Sum  Inputs=--++
  Constant : Constant  Value=0
  Demux : Demux
  Gain : Gain  Gain=-Ir
  Gain1 : Gain  Gain=Ir
  Multiply1 : Product
  Multiply2 : Product
  Mux : Mux  Inputs=3
  gyroscopic_torque : Outport  VectorParamsAs1DForOutWhenUnconnected=off
  wires:
  Add/1 -> Multiply2/1, Multiply1/1
  Demux/1 -> Add/1
  Multiply1/1 -> Gain/1
  Rotor_speed/1 -> Demux/1
  Demux/3 -> Add/3
  Demux/2 -> Add/2
  Demux/4 -> Add/4
  Multiply2/1 -> Gain1/1
  Gain1/1 -> Mux/2
  Mux/1 -> gyroscopic_torque/1
  Constant/1 -> Mux/3
  Gain/1 -> Mux/1
  p/1 -> Multiply2/2
  q/1 -> Multiply1/2

== system quadrotor/Motors & Propellers/Rotor_Generated_Torque ==
  Rotor_speed : Inport
  Multiply1 : Product  Multiplication=Matrix(*)
  Square1 : Math  Operator=square  SignedPower=on
  X_Frame : Constant  Value=[-LT*hT,LT*hT,LT*hT,-LT*hT;LT*hT,-LT*hT,LT*hT,-LT*hT;hM,hM,-hM,-hM]  OutDataTypeStr=double
  Torque : Outport  VectorParamsAs1DForOutWhenUnconnected=off
  wires:
  Square1/1 -> Multiply1/2
  Multiply1/1 -> Torque/1
  X_Frame/1 -> Multiply1/1
  Rotor_speed/1 -> Square1/1

== system quadrotor/Position & Velocity Control/Kd-vx ==
  evx : Inport
  Gain : Gain  Gain=kd_x
  kevx : Outport
  wires:
  evx/1 -> Gain/1
  Gain/1 -> kevx/1

== system quadrotor/Position & Velocity Control/Kd-vy ==
  evy : Inport
  Gain : Gain  Gain=kd_y
  kevy : Outport
  wires:
  evy/1 -> Gain/1
  Gain/1 -> kevy/1

== system quadrotor/Position & Velocity Control/Kd-vz ==
  evz : Inport
  Gain : Gain  Gain=kd_z
  kevz : Outport
  wires:
  evz/1 -> Gain/1
  Gain/1 -> kevz/1

== system quadrotor/Position & Velocity Control/Kp-x ==
  ex : Inport
  Gain : Gain  Gain=kp_x
  kex : Outport
  wires:
  ex/1 -> Gain/1
  Gain/1 -> kex/1

== system quadrotor/Position & Velocity Control/Kp-y ==
  ey : Inport
  Gain : Gain  Gain=kp_y
  key : Outport
  wires:
  ey/1 -> Gain/1
  Gain/1 -> key/1

== system quadrotor/Position & Velocity Control/Kp-z ==
  ez : Inport
  Gain : Gain  Gain=kp_z
  kez : Outport
  wires:
  Gain/1 -> kez/1
  ez/1 -> Gain/1  "ex"

== system quadrotor/Position & Velocity Control/Vx_PID ==
  In1 : Inport
  Derivative : Derivative  CoefficientInTFapproximation=T_d_v
  Gain6 : Gain  Gain=Kvx_P
  Gain7 : Gain  Gain=Kvx_I
  Gain8 : Gain  Gain=Kvx_D
  Integrator1 : Integrator  LimitOutput=on  UpperSaturationLimit=0.4  LowerSaturationLimit=-0.4
  Sum11 : Sum  Inputs=+++
  ux : Outport
  wires:
  Derivative/1 -> Sum11/3
  Gain8/1 -> Derivative/1
  Gain6/1 -> Sum11/2, Gain8/1, Gain7/1
  In1/1 -> Gain6/1  "ex"
  Integrator1/1 -> Sum11/1
  Gain7/1 -> Integrator1/1
  Sum11/1 -> ux/1

== system quadrotor/Position & Velocity Control/Vy_PID ==
  In1 : Inport
  Derivative : Derivative  CoefficientInTFapproximation=T_d_v
  Gain6 : Gain  Gain=Kvy_P
  Gain7 : Gain  Gain=Kvy_I
  Gain8 : Gain  Gain=Kvy_D
  Integrator1 : Integrator  LimitOutput=on  UpperSaturationLimit=0.4  LowerSaturationLimit=-0.4
  Sum11 : Sum  Inputs=+++
  ux : Outport
  wires:
  Derivative/1 -> Sum11/3
  Gain8/1 -> Derivative/1
  Gain6/1 -> Sum11/2, Gain8/1, Gain7/1
  In1/1 -> Gain6/1  "ex"
  Integrator1/1 -> Sum11/1
  Gain7/1 -> Integrator1/1
  Sum11/1 -> ux/1

== system quadrotor/Position & Velocity Control/Vz_PID ==
  In1 : Inport
  Derivative : Derivative  CoefficientInTFapproximation=T_d_v
  Gain6 : Gain  Gain=Kvz_P
  Gain7 : Gain  Gain=Kvz_I
  Gain8 : Gain  Gain=Kvz_D
  Integrator1 : Integrator  LimitOutput=on  UpperSaturationLimit=0.4  LowerSaturationLimit=-0.4
  Sum11 : Sum  Inputs=+++
  ux : Outport
  wires:
  Derivative/1 -> Sum11/3
  Gain8/1 -> Derivative/1
  Gain6/1 -> Sum11/2, Gain8/1, Gain7/1
  In1/1 -> Gain6/1  "ex"
  Integrator1/1 -> Sum11/1
  Gain7/1 -> Integrator1/1
  Sum11/1 -> ux/1

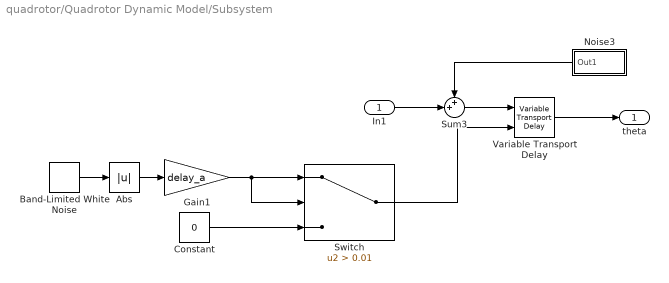
== system quadrotor/Quadrotor Dynamic Model/Subsystem ==
  In1 : Inport
  Abs : Abs  SaturateOnIntegerOverflow=off
  Band-Limited White Noise : simulink/Sources/Band-Limited White Noise  Cov=[0.05]  Ts=delay_sample  seed=[seed_delay_theta]
  Constant : Constant  Value=0
  Gain1 : Gain  Gain=delay_a
  Noise3 : Subsystem
  Sum3 : Sum  Inputs=++|
  Switch : Switch  Criteria=u2 > Threshold  Threshold=0.01  SaturateOnIntegerOverflow=off  InputSameDT=off
  Variable Transport Delay : VariableTransportDelay  MaximumDelay=delay_limit  ZeroDelay=on
  theta : Outport
  wires:
  Sum3/1 -> Variable Transport Delay/1
  Noise3/1(Out1) -> Sum3/1
  In1/1 -> Sum3/2
  Variable Transport Delay/1 -> theta/1
  Band-Limited White Noise/1 -> Abs/1
  Switch/1 -> Variable Transport Delay/2
  Abs/1 -> Gain1/1
  Constant/1 -> Switch/3
  Gain1/1 -> Switch/2, Switch/1

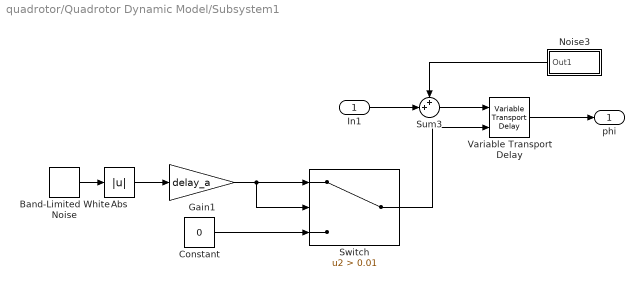
== system quadrotor/Quadrotor Dynamic Model/Subsystem1 ==
  In1 : Inport
  Abs : Abs  SaturateOnIntegerOverflow=off
  Band-Limited White Noise : simulink/Sources/Band-Limited White Noise  Cov=[0.05]  Ts=delay_sample  seed=[seed_delay_phi]
  Constant : Constant  Value=0
  Gain1 : Gain  Gain=delay_a
  Noise3 : Subsystem
  Sum3 : Sum  Inputs=++|
  Switch : Switch  Criteria=u2 > Threshold  Threshold=0.01  SaturateOnIntegerOverflow=off  InputSameDT=off
  Variable Transport Delay : VariableTransportDelay  MaximumDelay=delay_limit  ZeroDelay=on
  phi : Outport
  wires:
  Sum3/1 -> Variable Transport Delay/1
  Noise3/1(Out1) -> Sum3/1
  In1/1 -> Sum3/2
  Variable Transport Delay/1 -> phi/1
  Band-Limited White Noise/1 -> Abs/1
  Switch/1 -> Variable Transport Delay/2
  Abs/1 -> Gain1/1
  Constant/1 -> Switch/3
  Gain1/1 -> Switch/2, Switch/1

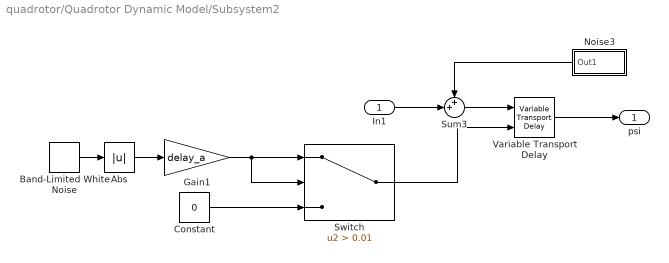
== system quadrotor/Quadrotor Dynamic Model/Subsystem2 ==
  In1 : Inport
  Abs : Abs  SaturateOnIntegerOverflow=off
  Band-Limited White Noise : simulink/Sources/Band-Limited White Noise  Cov=[0.05]  Ts=delay_sample  seed=[seed_delay_psi]
  Constant : Constant  Value=0
  Gain1 : Gain  Gain=delay_a
  Noise3 : Subsystem
  Sum3 : Sum  Inputs=++|
  Switch : Switch  Criteria=u2 > Threshold  Threshold=0.01  SaturateOnIntegerOverflow=off  InputSameDT=off
  Variable Transport Delay : VariableTransportDelay  MaximumDelay=delay_limit  ZeroDelay=on
  psi : Outport
  wires:
  Sum3/1 -> Variable Transport Delay/1
  Noise3/1(Out1) -> Sum3/1
  In1/1 -> Sum3/2
  Variable Transport Delay/1 -> psi/1
  Band-Limited White Noise/1 -> Abs/1
  Switch/1 -> Variable Transport Delay/2
  Abs/1 -> Gain1/1
  Gain1/1 -> Switch/2, Switch/1
  Constant/1 -> Switch/3

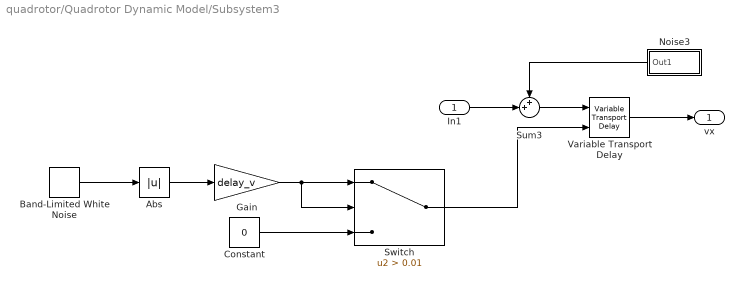
== system quadrotor/Quadrotor Dynamic Model/Subsystem3 ==
  In1 : Inport
  Abs : Abs  SaturateOnIntegerOverflow=off
  Band-Limited White Noise : simulink/Sources/Band-Limited White Noise  Cov=[0.05]  Ts=delay_sample  seed=[seed_delay_vx]
  Constant : Constant  Value=0
  Gain : Gain  Gain=delay_v
  Noise3 : Subsystem
  Sum3 : Sum  Inputs=++|
  Switch : Switch  Criteria=u2 > Threshold  Threshold=0.01  SaturateOnIntegerOverflow=off  InputSameDT=off
  Variable Transport Delay : VariableTransportDelay  MaximumDelay=delay_limit  ZeroDelay=on
  vx : Outport
  wires:
  Sum3/1 -> Variable Transport Delay/1
  Noise3/1(Out1) -> Sum3/1
  In1/1 -> Sum3/2
  Variable Transport Delay/1 -> vx/1
  Band-Limited White Noise/1 -> Abs/1
  Gain/1 -> Switch/2, Switch/1
  Abs/1 -> Gain/1
  Switch/1 -> Variable Transport Delay/2
  Constant/1 -> Switch/3

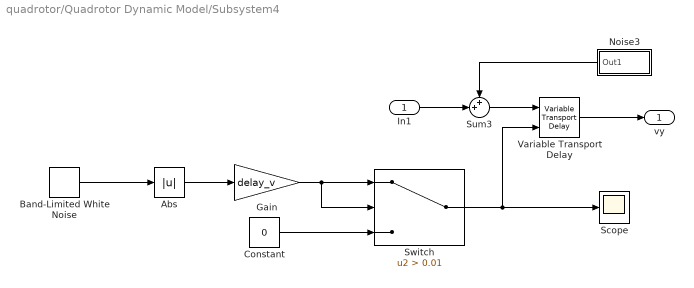
== system quadrotor/Quadrotor Dynamic Model/Subsystem4 ==
  In1 : Inport
  Abs : Abs  SaturateOnIntegerOverflow=off
  Band-Limited White Noise : simulink/Sources/Band-Limited White Noise  Cov=[0.05]  Ts=delay_sample  seed=[seed_delay_vy]
  Constant : Constant  Value=0
  Gain : Gain  Gain=delay_v
  Noise3 : Subsystem
  Scope : Scope
  Sum3 : Sum  Inputs=++|
  Switch : Switch  Criteria=u2 > Threshold  Threshold=0.01  SaturateOnIntegerOverflow=off  InputSameDT=off
  Variable Transport Delay : VariableTransportDelay  MaximumDelay=delay_limit  ZeroDelay=on
  vy : Outport
  wires:
  Sum3/1 -> Variable Transport Delay/1
  Noise3/1(Out1) -> Sum3/1
  In1/1 -> Sum3/2
  Variable Transport Delay/1 -> vy/1
  Band-Limited White Noise/1 -> Abs/1
  Switch/1 -> Scope/1, Variable Transport Delay/2
  Abs/1 -> Gain/1
  Gain/1 -> Switch/2, Switch/1
  Constant/1 -> Switch/3

== system quadrotor/Quadrotor Dynamic Model/Subsystem5 ==
  In1 : Inport
  Abs : Abs  SaturateOnIntegerOverflow=off
  Band-Limited White Noise : simulink/Sources/Band-Limited White Noise  Cov=[0.05]  Ts=delay_sample  seed=[seed_delay_vz]
  Constant : Constant  Value=0
  Gain : Gain  Gain=delay_v
  Noise3 : Subsystem
  Sum3 : Sum  Inputs=++|
  Switch : Switch  Criteria=u2 > Threshold  Threshold=0.01  SaturateOnIntegerOverflow=off  InputSameDT=off
  Variable Transport Delay : VariableTransportDelay  MaximumDelay=delay_limit  ZeroDelay=on
  vz : Outport
  wires:
  Sum3/1 -> Variable Transport Delay/1
  Noise3/1(Out1) -> Sum3/1
  In1/1 -> Sum3/2
  Variable Transport Delay/1 -> vz/1
  Band-Limited White Noise/1 -> Abs/1
  Abs/1 -> Gain/1
  Gain/1 -> Switch/2, Switch/1
  Constant/1 -> Switch/3
  Switch/1 -> Variable Transport Delay/2

== system quadrotor/Quadrotor Dynamic Model/Subsystem/Noise3 ==
  Band-Limited White Noise : simulink/Sources/Band-Limited White Noise  Cov=1  Ts=sample_a  seed=[seed_theta]
  Gain : Gain  Gain=noise_a
  Out1 : Outport
  wires:
  Band-Limited White Noise/1 -> Gain/1
  Gain/1 -> Out1/1

== system quadrotor/Quadrotor Dynamic Model/Subsystem1/Noise3 ==
  Band-Limited White Noise : simulink/Sources/Band-Limited White Noise  Cov=1  Ts=sample_a  seed=[seed_phi]
  Gain : Gain  Gain=noise_a
  Out1 : Outport
  wires:
  Band-Limited White Noise/1 -> Gain/1
  Gain/1 -> Out1/1

== system quadrotor/Quadrotor Dynamic Model/Subsystem2/Noise3 ==
  Band-Limited White Noise : simulink/Sources/Band-Limited White Noise  Cov=1  Ts=sample_a  seed=[seed_psi]
  Gain : Gain  Gain=noise_a
  Out1 : Outport
  wires:
  Band-Limited White Noise/1 -> Gain/1
  Gain/1 -> Out1/1

== system quadrotor/Quadrotor Dynamic Model/Subsystem3/Noise3 ==
  Band-Limited White Noise : simulink/Sources/Band-Limited White Noise  Cov=1  Ts=sample_v  seed=[seed_vx]
  Gain : Gain  Gain=noise_v
  Out1 : Outport
  wires:
  Band-Limited White Noise/1 -> Gain/1
  Gain/1 -> Out1/1

== system quadrotor/Quadrotor Dynamic Model/Subsystem4/Noise3 ==
  Band-Limited White Noise : simulink/Sources/Band-Limited White Noise  Cov=1  Ts=sample_v  seed=[seed_vy]
  Gain : Gain  Gain=noise_v
  Out1 : Outport
  wires:
  Band-Limited White Noise/1 -> Gain/1
  Gain/1 -> Out1/1

== system quadrotor/Quadrotor Dynamic Model/Subsystem5/Noise3 ==
  Band-Limited White Noise : simulink/Sources/Band-Limited White Noise  Cov=1  Ts=sample_v  seed=[seed_vz]
  Gain : Gain  Gain=noise_v
  Out1 : Outport
  wires:
  Band-Limited White Noise/1 -> Gain/1
  Gain/1 -> Out1/1

== matlab function quadrotor/Quadrotor Dynamic Model/dw//dt ==
  data: u input; v input; w input; dw output; p input; q input; theta input; phi input; CDz input; f_zb input; T input; g input; m input
function dw = Equation_dw(u,v,w,p,q,theta,phi,CDz,f_zb,T,g,m)
dw = u*q - v*p + g*cos(theta)*cos(phi) - T/m - CDz*w*abs(w)/m + f_zb/m;
end

== matlab function quadrotor/Quadrotor Dynamic Model/dp//dt ==
  data: q input; r input; Ix input; Iy input; Iz input; gyroeffect_xb input; dp output; tau_xb input; ftau_xb input
function dp = Equation_dp(q,r,Ix,Iy,Iz,gyroeffect_xb,tau_xb,ftau_xb)
dp = (q*r*(Iy-Iz) + gyroeffect_xb + tau_xb + ftau_xb)/Ix;
end

== matlab function quadrotor/Quadrotor Dynamic Model/dq//dt ==
  data: p input; r input; Ix input; Iy input; Iz input; gyroeffect_yb input; dq output; tau_yb input; ftau_yb input
function dq = Equation_dq(p,r,Ix,Iy,Iz,gyroeffect_yb,tau_yb,ftau_yb)
dq = (p*r*(Iz-Ix)+ gyroeffect_yb + tau_yb + ftau_yb)/Iy;
end

== matlab function quadrotor/Quadrotor Dynamic Model/dr//dt ==
  data: p input; q input; Ix input; Iy input; Iz input; gyroeffect_zb input; tau_zb input; dr output; ftau_zb input
function dr = Equation_dr(p,q,Ix,Iy,Iz,gyroeffect_zb,tau_zb,ftau_zb)
dr = (p*q*(Ix-Iy) + gyroeffect_zb + tau_zb + ftau_zb)/Iz;
end

== matlab function quadrotor/Quadrotor Dynamic Model/dtheta//dt ==
  data: q input; r input; phi input; dtheta output
function dtheta = Equation_dtheta(q,r,phi)
dtheta = q*cos(phi) - r*sin(phi);
end

== matlab function quadrotor/Quadrotor Dynamic Model/dpsi//dt ==
  data: q input; r input; theta input; phi input; dpsi output
function dpsi = Equation_dpsi(q,r,theta,phi)
dpsi = (r*cos(phi)+q*sin(phi))/cos(theta);
end

== matlab function quadrotor/Quadrotor Dynamic Model/Coordinate Transformation Ground-frame to Body-frame ==
  data: xg input; yg input; zg input; xb output; yb output; zb output; theta input; phi input; psi input
% ==== coordinate transformation function ====
% 
% ==== variables ====
% theta,phi,psi - Euler angles 
% Vg=[xg;yg;zg] - vector in ground coordinate
% Vb=[xb;yb;zb] - vector in body coordinate
% 
% ==== function ====
% This function transfers Vb to Vg.
% 
% ===== note =====
% 


function [xb,yb,zb] = G_to_B(xg,yg,zg,theta,phi,psi)
  S_trans = zeros(3,3);
  S_trans(1,:) = [cos(psi)*cos(theta), cos(psi)*sin(theta)*sin(phi)-cos(phi)*sin(psi), sin(psi)*sin(phi)+cos(psi)*cos(phi)*sin(theta)];
  S_trans(2,:) = [cos(theta)*sin(psi), cos(psi)*cos(phi)+sin(psi)*sin(theta)*sin(phi), cos(phi)*sin(psi)*sin(theta)-cos(psi)*sin(phi)];
  S_trans(3,:) = [-sin(theta), cos(theta)*sin(phi), cos(theta)*cos(phi)];
  S_trans = S_trans';
  xb = S_trans(1,:)*[xg;yg;zg];
  yb = S_trans(2,:)*[xg;yg;zg];
  zb = S_trans(3,:)*[xg;yg;zg];
end

== matlab function quadrotor/Quadrotor Dynamic Model/Coordinate Transformation Body-frame to Ground-frame ==
  data: xg output; yg output; zg output; xb input; yb input; zb input; theta input; phi input; psi input
% ==== coordinate transformation function ====
% 
% ==== variables ====
% theta,phi,psi - Euler angles 
% Vg=[xg;yg;zg] - vector in ground coordinate
% Vb=[xb;yb;zb] - vector in body coordinate
% 
% ==== function ====
% This function transfers Vb to Vg.
% 
% ===== note =====
% 


function [xg,yg,zg] = B_to_G(xb,yb,zb,theta,phi,psi)
  S_trans = zeros(3,3);
  S_trans(1,:) = [cos(psi)*cos(theta), cos(psi)*sin(theta)*sin(phi)-cos(phi)*sin(psi), sin(psi)*sin(phi)+cos(psi)*sin(theta)*cos(phi)];
  S_trans(2,:) = [cos(theta)*sin(psi), cos(psi)*cos(phi)+sin(psi)*sin(theta)*sin(phi), sin(psi)*cos(phi)*sin(theta)-cos(psi)*sin(phi)];
  S_trans(3,:) = [-sin(theta), cos(theta)*sin(phi), cos(theta)*cos(phi)];
  xg = S_trans(1,:)*[xb;yb;zb];
  yg = S_trans(2,:)*[xb;yb;zb];
  zg = S_trans(3,:)*[xb;yb;zb];
end

== matlab function quadrotor/Position & Velocity Control/MATLAB Function ==
  data: ux input; psi input; phi output; uy input; theta output
function [phi, theta] = fcn(ux, psi, uy)
phi = sin(psi)*ux - cos(psi)*uy;
theta = cos(psi)*ux - sin(psi)*uy;

== matlab function quadrotor/Quadrotor Dynamic Model/dphi//dt ==
  data: p input; q input; r input; theta input; phi input; dphi output
function dphi = Equation_dphi(p,q,r,theta,phi)
dphi = p + (r*cos(phi)+q*sin(phi))*tan(theta);
end

== matlab function quadrotor/Quadrotor Dynamic Model/du//dt ==
  data: u input; v input; w input; du output; q input; r input; theta input; CDx input; f_xb input; g input; m input
function du = Equation_du(u,v,w,q,r,theta,CDx,f_xb,g,m)
du = v*r - w*q - g*sin(theta) - CDx*u*abs(u)/m + f_xb/m;
% - CDx*u*abs(u) is the air drag along body-x axis
end

== matlab function quadrotor/Quadrotor Dynamic Model/dv//dt ==
  data: u input; v input; w input; dv output; p input; r input; theta input; phi input; CDy input; f_yb input; g input; m input
function dv = Equation_dv(u,v,w,p,r,theta,phi,CDy,f_yb,g,m)
dv = -u*r + w*p + g*cos(theta)*sin(phi) - CDy*v*abs(v)/m + f_yb/m;
end
